simulink model "ResourceProcessor"  (R2023b)
settings: Solver=VariableStepAuto  StartTime=0.0  StopTime=10.0  RelTol=1e-3
settings Model: Creator=user  LastModifiedBy=user

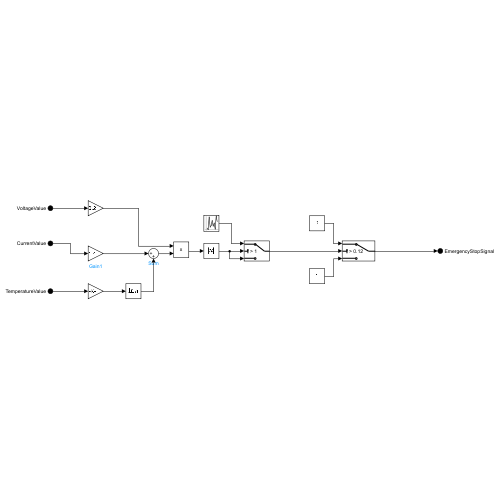
[thumbnail: Simulink's stored preview of the top-level diagram]
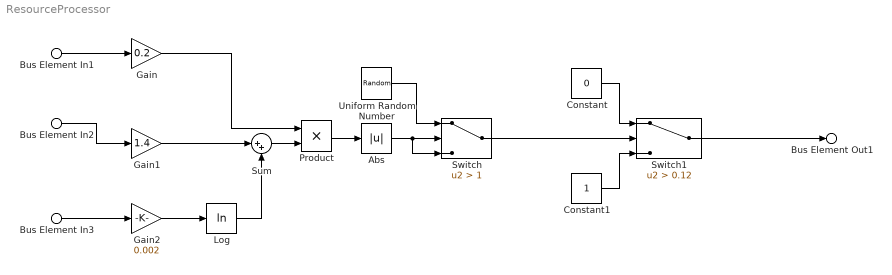
== system ResourceProcessor ==
  Bus Element In1 : Inport  PortName=VoltageValue
  Bus Element In2 : Inport  Port=2  PortName=CurrentValue
  Bus Element In3 : Inport  Port=3  PortName=TemperatureValue
  Abs : Abs  SaturateOnIntegerOverflow=off
  Constant : Constant  Value=0
  Constant1 : Constant
  Gain : Gain  Gain=0.2
  Gain1 : Gain  Gain=1.4
  Gain2 : Gain  Gain=0.002
  Log : Math  Operator=log
  Product : Product
  Sum : Sum  Inputs=|++
  Switch : Switch  Criteria=u2 > Threshold  Threshold=1  SaturateOnIntegerOverflow=off  InputSameDT=off
  Switch1 : Switch  Criteria=u2 > Threshold  Threshold=0.12  SaturateOnIntegerOverflow=off  InputSameDT=off
  Uniform Random Number : UniformRandomNumber  SampleTime=0.1
  Bus Element Out1 : Outport  PortName=EmergencyStopSignal
  wires:
  Gain2/1 -> Log/1
  Gain1/1 -> Sum/1
  Log/1 -> Sum/2
  Sum/1 -> Product/2
  Gain/1 -> Product/1
  Bus Element In1/1 -> Gain/1
  Bus Element In2/1 -> Gain1/1
  Bus Element In3/1 -> Gain2/1
  Product/1 -> Abs/1
  Abs/1 -> Switch/3, Switch/2
  Uniform Random Number/1 -> Switch/1
  Switch/1 -> Switch1/2
  Switch1/1 -> Bus Element Out1/1
  Constant/1 -> Switch1/1
  Constant1/1 -> Switch1/3
